simulink model "pwm"  (R2014a)
settings: Solver=ode45  StartTime=0.0  StopTime=10.0  RelTol=1e-3
settings Model: Creator=RANGA  LastModifiedBy=RANGA

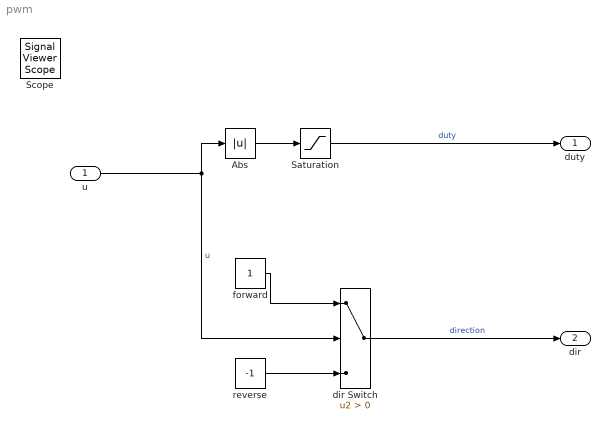
== system pwm ==
  u : Inport
  Abs : Abs
  Saturation : Saturate  UpperLimit=1  LowerLimit=0
  dir Switch : Switch  Criteria=u2 > Threshold
  forward : Constant
  reverse : Constant  Value=-1
  duty : Outport
  dir : Outport  Port=2
  Scope : SignalViewerScope  IOType=viewer  NumInputPorts=3  RefreshTime=0.035000
      settings: YMin=-5~-5~-5  YMax=5~5~5
  wires:
  forward/1 -> dir Switch/1
  u/1 -> Abs/1, dir Switch/2  "u"
  reverse/1 -> dir Switch/3
  Abs/1 -> Saturation/1
  dir Switch/1 -> dir/1  "direction"
  Saturation/1 -> duty/1  "duty"
